simulink model "concatdoc"  (Simulink 5.0)
settings: Solver=ode45  SolverMode=SingleTasking  StartTime=0.0  StopTime=inf  RelTol=1e-3
undefined symbols (not defined in the file or in its folder): EbNodB, M, rsgenpoly, slcm
libraries: commutil2 x3, dspsigops x3, commcnvcod2 x2, commsink2 x2, commsequence2 x2, commblkcod2 x2, commchan2 x1, commrandsrc2 x1
settings Model: Creator=agaltman  LastModifiedBy=agaltman  SaveTime=off  SaveOutput=off  SignalLoggingName=logsOut  AlgebraicLoopMsg=error  RTWInlineParameters=on  BooleanDataType=off  ZeroCrossControl=UseLocalSettings  RTWMathFcnLibMatFile=iso_c_tmw.mat  RTWOptions=-aRollThreshold=5

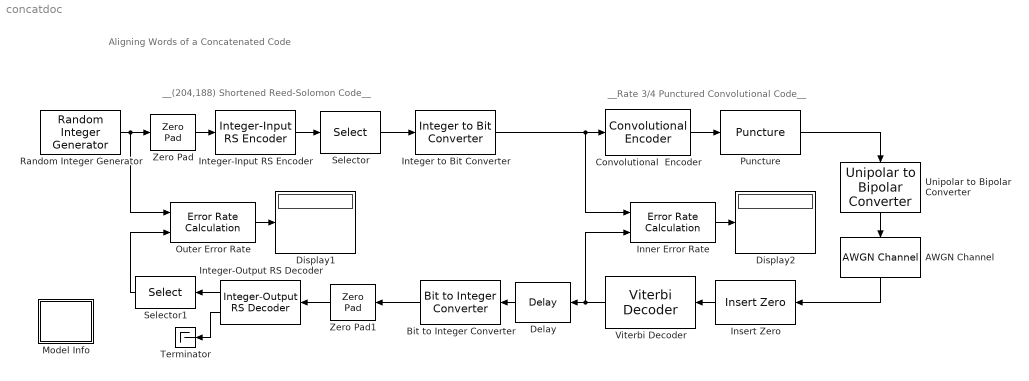
== system concatdoc ==
  note: __(204,188) Shortened Reed-Solomon Code__
  note: __Rate 3/4 Punctured Convolutional Code__
  note: Aligning Words of a Concatenated Code
  AWGN Channel : commchan2/AWGN Channel  Orientation=down  seed=68521  noiseMode="Signal to noise ratio  (SNR)"  EsNodB=EbNodB+10*log10(log2(M))  SNRdB=5  Ps=1  Tsym=Tsym  variance=10^(-0.1*15)/(2048*2)
  Bit to Integer Converter : commutil2/Bit to Integer Converter  Orientation=left  nbits=8
  Convolutional  Encoder : commcnvcod2/Convolutional Encoder  trellis=poly2trellis(7, [171 133])  reset=None
  Delay : dspsigops/Delay  Orientation=left  dly_unit=Samples  delay=1632-136  ic_detail=off  dif_ic_for_ch=off  dif_ic_for_dly=off  ic=0  reset_popup=None
  Display1 : Display
  Display2 : Display
  Inner Error Rate : commsink2/Error Rate Calculation  N=136  st_delay=0  cp_mode=Entire frame  subframe=[]  PMode=Port  WsName=ErrorVec  RsMode2=off  stop=on  numErr=100  maxBits=1e6
  Insert Zero : commsequence2/Insert Zero  Orientation=left  insertZeroVector=[1 1 0 1 1 0]'
  Integer to Bit Converter : commutil2/Integer to Bit Converter  nbits=8
  Integer-Input RS Encoder : commblkcod2/Integer-Input RS Encoder  n=255  k=239  specPrimPoly=off  primPoly=[1 0 1 1]  specGenPoly=off  genPoly=rsgenpoly(7,3)
  Integer-Output RS Decoder : commblkcod2/Integer-Output RS Decoder  Orientation=left  n=255  k=239  specPrimPoly=off  primPoly=[1 0 1 1]  specGenPoly=off  genPoly=rsgenpoly(7,3)  showNumErr=on
  Model Info : Subsystem  LoadFcn=slcm LoadBlock;  InitFcn=slcm('UpdateAllCMBlocksInThisModelInit')  mask(CMBlock){InitialSaveTempField=, InitialBlockCM=None, BlockCM=None, Frame=on, SaveTempField=, DisplayStringWithTags=Info, MaskDisplayString=Info, HorizontalTextAlignment=Center, LeftAlignmentValue=0.5, SourceBlockDiagram=concatdoc, TagMaxNumber=20, CMTag1=, CMTag2=, CMTag3=, CMTag4=, CMTag5=, CMTag6=, CMTag7=, CMTag8=, CMTag9=, CMTag10=, CMTag11=, CMTag12=, CMTag13=, CMTag14=, CMTag15=, CMTag16=, CMTag17=, CMTag18=, CMTag19=, CMTag20=}
      mask help: This block allows revision control information to be displayed within the model.
      settings: CopyFcn=slcm CopyBlock;  DeleteFcn=slcm Cancel;  PostSaveFcn=slcm('UpdateAllCMBlocksInThisModel')  NameChangeFcn=slcm Rename;  OpenFcn=commdemohelp;
      mask Display: text(str2num(LeftAlignmentValue), 0.5, MaskDisplayString, 'HorizontalAlignment', HorizontalTextAlignment)
  Outer Error Rate : commsink2/Error Rate Calculation  N=188  st_delay=0  cp_mode=Entire frame  subframe=[]  PMode=Port  WsName=ErrorVec  RsMode2=off  stop=off  numErr=100  maxBits=1e6
  Puncture : commsequence2/Puncture  punctureVector=[1 1 0 1 1 0]'
  Random Integer Generator : commrandsrc2/Random Integer Generator  mul=256  seed=56479  Ts=1  frameBased=on  sampPerFrame=188  orient=off
  Selector : Selector  Elements=[1:204]  InputPortWidth=255
  Selector1 : Selector  Orientation=left  Elements=[1:188]  InputPortWidth=239
  Terminator : Terminator
  Unipolar to Bipolar Converter : commutil2/Unipolar to Bipolar Converter  Orientation=down  M=2  polarity=Negative
  Viterbi Decoder : commcnvcod2/Viterbi Decoder  Orientation=left  trellis=poly2trellis(7, [171 133])  dectype=Unquantized  nsdecb=4  tbdepth=136  opmode=Continuous  reset=off
  Zero Pad : dspsigops/Zero Pad  padSigAt=End  zpadAlong=Columns  padNumOutRowsSpecMethod=User-specified  numOutRows=239  padNumOutColsSpecMethod=User-specified  numOutCols=1  trunc_flag=None
  Zero Pad1 : dspsigops/Zero Pad  Orientation=left  padSigAt=End  zpadAlong=Columns  padNumOutRowsSpecMethod=User-specified  numOutRows=255  padNumOutColsSpecMethod=User-specified  numOutCols=1  trunc_flag=None
  wires:
  Random Integer Generator/1 -> Zero Pad/1, Outer Error Rate/1
  Zero Pad/1 -> Integer-Input RS Encoder/1
  Integer-Input RS Encoder/1 -> Selector/1
  Selector/1 -> Integer to Bit Converter/1
  Integer to Bit Converter/1 -> Inner Error Rate/1, Convolutional  Encoder/1
  Convolutional  Encoder/1 -> Puncture/1
  Puncture/1 -> Unipolar to Bipolar Converter/1
  Viterbi Decoder/1 -> Inner Error Rate/2, Delay/1
  Bit to Integer Converter/1 -> Zero Pad1/1
  Zero Pad1/1 -> Integer-Output RS Decoder/1
  Integer-Output RS Decoder/1 -> Selector1/1
  Integer-Output RS Decoder/2 -> Terminator/1
  Selector1/1 -> Outer Error Rate/2
  Outer Error Rate/1 -> Display1/1
  Inner Error Rate/1 -> Display2/1
  Insert Zero/1 -> Viterbi Decoder/1
  Unipolar to Bipolar Converter/1 -> AWGN Channel/1
  Delay/1 -> Bit to Integer Converter/1
  AWGN Channel/1 -> Insert Zero/1

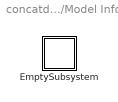
== system concatdoc/Model Info ==
  EmptySubsystem : Subsystem

== system concatdoc/Model Info/EmptySubsystem ==
